simulink model "case8"  (R2024b)
settings: Solver=FixedStepAuto  StartTime=0  StopTime=1  FixedStep=1e-7  RelTol=1e-3
values from neighbouring files (symbols this model uses):
  SG_D_1_D = 0.01056    [IEEE9_case_parameters.m]    (also in case1_parameters.m; case2_parameters.m; case3_parameters.m; case4_parameters.m)
  SG_D_1_EnableSaturation = 0    [IEEE9_case_parameters.m]    (also in case1_parameters.m; case2_parameters.m; case3_parameters.m; case4_parameters.m)
  SG_D_1_f0 = 60    [IEEE9_case_parameters.m]    (also in case1_parameters.m; case2_parameters.m; case3_parameters.m; case4_parameters.m)
  SG_D_1_H = 7.5    [IEEE9_case_parameters.m]    (also in case1_parameters.m; case2_parameters.m; case3_parameters.m; case4_parameters.m)
  SG_D_1_K_A = 20    [IEEE9_case_parameters.m]    (also in case1_parameters.m; case2_parameters.m; case3_parameters.m; case4_parameters.m)
  SG_D_1_K_E = 1.000000e+1    (= 10)    [IEEE9_case_parameters.m]    (also in case1_parameters.m; case2_parameters.m; case3_parameters.m; case4_parameters.m)
  SG_D_1_K_F = 2.363    [IEEE9_case_parameters.m]    (also in case1_parameters.m; case2_parameters.m; case3_parameters.m; case4_parameters.m)
  SG_D_1_K_s = 0.5    [IEEE9_case_parameters.m]    (also in case1_parameters.m = 5; case2_parameters.m = 5; case3_parameters.m = 5; case4_parameters.m = 5)
  SG_D_1_R_a = 0.001088    [IEEE9_case_parameters.m]    (also in case1_parameters.m; case2_parameters.m; case3_parameters.m; case4_parameters.m)
  SG_D_1_S_A = 1    [IEEE9_case_parameters.m]    (also in case1_parameters.m; case2_parameters.m; case3_parameters.m; case4_parameters.m)
  SG_D_1_S_B = 0.103    [IEEE9_case_parameters.m]    (also in case1_parameters.m; case2_parameters.m; case3_parameters.m; case4_parameters.m)
  SG_D_1_S_N = 10.659857    [IEEE9_case_parameters.m]    (also in case1_parameters.m; case2_parameters.m; case3_parameters.m; case4_parameters.m)
  SG_D_1_SpeedPara = 200    [IEEE9_case_parameters.m]    (also in case1_parameters.m; case2_parameters.m; case3_parameters.m; case4_parameters.m)
  SG_D_1_T_0 = 0.720173    [IEEE9_case_parameters.m]    (also in case1_parameters.m = 0.755522; case2_parameters.m = 0.808931; case3_parameters.m = 0.869402; case4_parameters.m = 0.729316)
  SG_D_1_T_1 = 0.3    [IEEE9_case_parameters.m]    (also in case1_parameters.m; case2_parameters.m; case3_parameters.m; case4_parameters.m)
  SG_D_1_T_2 = 0.05    [IEEE9_case_parameters.m]    (also in case1_parameters.m; case2_parameters.m; case3_parameters.m; case4_parameters.m)
  SG_D_1_T_3 = 0.02    [IEEE9_case_parameters.m]    (also in case1_parameters.m; case2_parameters.m; case3_parameters.m; case4_parameters.m)
  SG_D_1_T_4 = 0.005    [IEEE9_case_parameters.m]    (also in case1_parameters.m; case2_parameters.m; case3_parameters.m; case4_parameters.m)
  SG_D_1_T_A = 0.02    [IEEE9_case_parameters.m]    (also in case1_parameters.m; case2_parameters.m; case3_parameters.m; case4_parameters.m)
  SG_D_1_T_dd = 8.000000e+0    (= 8)    [IEEE9_case_parameters.m]    (also in case1_parameters.m; case2_parameters.m; case3_parameters.m; case4_parameters.m)
  SG_D_1_T_ddd = 0.04    [IEEE9_case_parameters.m]    (also in case1_parameters.m; case2_parameters.m; case3_parameters.m; case4_parameters.m)
  SG_D_1_T_E = 0.314    [IEEE9_case_parameters.m]    (also in case1_parameters.m; case2_parameters.m; case3_parameters.m; case4_parameters.m)
  SG_D_1_T_F = 0.35    [IEEE9_case_parameters.m]    (also in case1_parameters.m; case2_parameters.m; case3_parameters.m; case4_parameters.m)
  SG_D_1_T_qd = 0.8    [IEEE9_case_parameters.m]    (also in case1_parameters.m; case2_parameters.m; case3_parameters.m; case4_parameters.m)
  SG_D_1_T_qdd = 0.02    [IEEE9_case_parameters.m]    (also in case1_parameters.m; case2_parameters.m; case3_parameters.m; case4_parameters.m)
  SG_D_1_T_speed = 0.1    [IEEE9_case_parameters.m]    (also in case1_parameters.m = 200; case2_parameters.m = 200; case3_parameters.m = 200; case4_parameters.m = 200)
  SG_D_1_T_w = 0.5    [IEEE9_case_parameters.m]    (also in case1_parameters.m; case2_parameters.m; case3_parameters.m; case4_parameters.m)
  SG_D_1_V_ref = 1.990276    [IEEE9_case_parameters.m]    (also in case1_parameters.m = 2.042296; case2_parameters.m = 2.051388; case3_parameters.m = 2.089584; case4_parameters.m = 2.01845)
  SG_D_1_w_ref = 376.991118    [IEEE9_case_parameters.m]    (also in case1_parameters.m; case2_parameters.m; case3_parameters.m; case4_parameters.m)
  SG_D_1_wb = 6.000000e+1    (= 60)    [IEEE9_case_parameters.m]    (also in case1_parameters.m; case2_parameters.m; case3_parameters.m; case4_parameters.m)
  SG_D_1_x_d = 1.9    [IEEE9_case_parameters.m]    (also in case1_parameters.m; case2_parameters.m; case3_parameters.m; case4_parameters.m)
  SG_D_1_x_dd = 0.302    [IEEE9_case_parameters.m]    (also in case1_parameters.m; case2_parameters.m; case3_parameters.m; case4_parameters.m)
  SG_D_1_x_ddd = 0.204    [IEEE9_case_parameters.m]    (also in case1_parameters.m; case2_parameters.m; case3_parameters.m; case4_parameters.m)
  SG_D_1_x_l = 0.05    [IEEE9_case_parameters.m]    (also in case1_parameters.m; case2_parameters.m; case3_parameters.m; case4_parameters.m)
  SG_D_1_x_q = 1.3    [IEEE9_case_parameters.m]    (also in case1_parameters.m; case2_parameters.m; case3_parameters.m; case4_parameters.m)
  SG_D_1_x_qd = 0.5    [IEEE9_case_parameters.m]    (also in case1_parameters.m; case2_parameters.m; case3_parameters.m; case4_parameters.m)
  SG_D_1_x_qdd = 0.3    [IEEE9_case_parameters.m]    (also in case1_parameters.m; case2_parameters.m; case3_parameters.m; case4_parameters.m)
  SG_D_2_D = 0.02    [IEEE9_case_parameters.m]    (also in case1_parameters.m; case2_parameters.m; case3_parameters.m; case4_parameters.m)
  SG_D_2_EnableSaturation = 0    [IEEE9_case_parameters.m]    (also in case1_parameters.m; case2_parameters.m; case3_parameters.m; case4_parameters.m)
  SG_D_2_f0 = 60    [IEEE9_case_parameters.m]    (also in case1_parameters.m; case2_parameters.m; case3_parameters.m; case4_parameters.m)
  SG_D_2_H = 8.000000e+0    (= 8)    [IEEE9_case_parameters.m]    (also in case1_parameters.m; case2_parameters.m; case3_parameters.m; case4_parameters.m)
  SG_D_2_K_A = 20    [IEEE9_case_parameters.m]    (also in case1_parameters.m; case2_parameters.m; case3_parameters.m; case4_parameters.m)
  SG_D_2_K_E = 1.000000e+1    (= 10)    [IEEE9_case_parameters.m]    (also in case1_parameters.m; case2_parameters.m; case3_parameters.m; case4_parameters.m)
  SG_D_2_K_F = 2.363    [IEEE9_case_parameters.m]    (also in case1_parameters.m; case2_parameters.m; case3_parameters.m; case4_parameters.m)
  SG_D_2_K_s = 0.5    [IEEE9_case_parameters.m]    (also in case1_parameters.m = 4; case2_parameters.m = 4; case3_parameters.m = 4; case4_parameters.m = 4)
  SG_D_2_R_a = 0.001088    [IEEE9_case_parameters.m]    (also in case1_parameters.m; case2_parameters.m; case3_parameters.m; case4_parameters.m)
  SG_D_2_S_A = 1    [IEEE9_case_parameters.m]    (also in case1_parameters.m; case2_parameters.m; case3_parameters.m; case4_parameters.m)
  SG_D_2_S_B = 0.103    [IEEE9_case_parameters.m]    (also in case1_parameters.m; case2_parameters.m; case3_parameters.m; case4_parameters.m)
  SG_D_2_S_N = 10.659857    [IEEE9_case_parameters.m]    (also in case1_parameters.m; case2_parameters.m; case3_parameters.m; case4_parameters.m)
  SG_D_2_SpeedPara = 200    [IEEE9_case_parameters.m]    (also in case1_parameters.m; case2_parameters.m; case3_parameters.m; case4_parameters.m)
  SG_D_2_T_0 = 1.632913    [IEEE9_case_parameters.m]    (also in case1_parameters.m = 1.632925; case2_parameters.m = 1.632915; case3_parameters.m = 1.632914; case4_parameters.m = 1.632927)
  SG_D_2_T_1 = 0.2    [IEEE9_case_parameters.m]    (also in case1_parameters.m; case2_parameters.m; case3_parameters.m; case4_parameters.m)
  SG_D_2_T_2 = 0.05    [IEEE9_case_parameters.m]    (also in case1_parameters.m; case2_parameters.m; case3_parameters.m; case4_parameters.m)
  SG_D_2_T_3 = 0.02    [IEEE9_case_parameters.m]    (also in case1_parameters.m; case2_parameters.m; case3_parameters.m; case4_parameters.m)
  SG_D_2_T_4 = 0.005    [IEEE9_case_parameters.m]    (also in case1_parameters.m; case2_parameters.m; case3_parameters.m; case4_parameters.m)
  SG_D_2_T_A = 0.02    [IEEE9_case_parameters.m]    (also in case1_parameters.m; case2_parameters.m; case3_parameters.m; case4_parameters.m)
  SG_D_2_T_dd = 7.9    [IEEE9_case_parameters.m]    (also in case1_parameters.m; case2_parameters.m; case3_parameters.m; case4_parameters.m)
  SG_D_2_T_ddd = 0.04    [IEEE9_case_parameters.m]    (also in case1_parameters.m; case2_parameters.m; case3_parameters.m; case4_parameters.m)
  SG_D_2_T_E = 0.314    [IEEE9_case_parameters.m]    (also in case1_parameters.m; case2_parameters.m; case3_parameters.m; case4_parameters.m)
  SG_D_2_T_F = 0.35    [IEEE9_case_parameters.m]    (also in case1_parameters.m; case2_parameters.m; case3_parameters.m; case4_parameters.m)
  SG_D_2_T_qd = 0.8    [IEEE9_case_parameters.m]    (also in case1_parameters.m; case2_parameters.m; case3_parameters.m; case4_parameters.m)
  SG_D_2_T_qdd = 0.015    [IEEE9_case_parameters.m]    (also in case1_parameters.m; case2_parameters.m; case3_parameters.m; case4_parameters.m)
  SG_D_2_T_speed = 0.1    [IEEE9_case_parameters.m]    (also in case1_parameters.m = 150; case2_parameters.m = 150; case3_parameters.m = 150; case4_parameters.m = 150)
  SG_D_2_T_w = 0.35    [IEEE9_case_parameters.m]    (also in case1_parameters.m; case2_parameters.m; case3_parameters.m; case4_parameters.m)
  SG_D_2_V_ref = 2.58547    [IEEE9_case_parameters.m]    (also in case1_parameters.m = 2.597896; case2_parameters.m = 2.587136; case3_parameters.m = 2.586042; case4_parameters.m = 2.599679)
  SG_D_2_w_ref = 376.991118    [IEEE9_case_parameters.m]    (also in case1_parameters.m; case2_parameters.m; case3_parameters.m; case4_parameters.m)
  SG_D_2_wb = 6.000000e+1    (= 60)    [IEEE9_case_parameters.m]    (also in case1_parameters.m; case2_parameters.m; case3_parameters.m; case4_parameters.m)
  SG_D_2_x_d = 1.8    [IEEE9_case_parameters.m]    (also in case1_parameters.m; case2_parameters.m; case3_parameters.m; case4_parameters.m)
  SG_D_2_x_dd = 0.302    [IEEE9_case_parameters.m]    (also in case1_parameters.m; case2_parameters.m; case3_parameters.m; case4_parameters.m)
  SG_D_2_x_ddd = 0.204    [IEEE9_case_parameters.m]    (also in case1_parameters.m; case2_parameters.m; case3_parameters.m; case4_parameters.m)
  SG_D_2_x_l = 0.05    [IEEE9_case_parameters.m]    (also in case1_parameters.m; case2_parameters.m; case3_parameters.m; case4_parameters.m)
  SG_D_2_x_q = 1.25    [IEEE9_case_parameters.m]    (also in case1_parameters.m; case2_parameters.m; case3_parameters.m; case4_parameters.m)
  SG_D_2_x_qd = 0.5    [IEEE9_case_parameters.m]    (also in case1_parameters.m; case2_parameters.m; case3_parameters.m; case4_parameters.m)
  SG_D_2_x_qdd = 0.3    [IEEE9_case_parameters.m]    (also in case1_parameters.m; case2_parameters.m; case3_parameters.m; case4_parameters.m)
  SG_D_3_D = 0.02    [IEEE9_case_parameters.m]    (also in case1_parameters.m; case2_parameters.m; case3_parameters.m; case4_parameters.m)
  SG_D_3_EnableSaturation = 0    [IEEE9_case_parameters.m]    (also in case1_parameters.m; case2_parameters.m; case3_parameters.m; case4_parameters.m)
  SG_D_3_f0 = 60    [IEEE9_case_parameters.m]    (also in case1_parameters.m; case2_parameters.m; case3_parameters.m; case4_parameters.m)
  SG_D_3_H = 7.7    [IEEE9_case_parameters.m]    (also in case1_parameters.m; case2_parameters.m; case3_parameters.m; case4_parameters.m)
  SG_D_3_K_A = 20    [IEEE9_case_parameters.m]    (also in case1_parameters.m; case2_parameters.m; case3_parameters.m; case4_parameters.m)
  SG_D_3_K_E = 1.000000e+1    (= 10)    [IEEE9_case_parameters.m]    (also in case1_parameters.m; case2_parameters.m; case3_parameters.m; case4_parameters.m)
  SG_D_3_K_F = 2.363    [IEEE9_case_parameters.m]    (also in case1_parameters.m; case2_parameters.m; case3_parameters.m; case4_parameters.m)
  SG_D_3_K_s = 0.2    [IEEE9_case_parameters.m]    (also in case1_parameters.m = 2; case2_parameters.m = 2; case3_parameters.m = 2; case4_parameters.m = 2)
  SG_D_3_R_a = 0.001088    [IEEE9_case_parameters.m]    (also in case1_parameters.m; case2_parameters.m; case3_parameters.m; case4_parameters.m)
  SG_D_3_S_A = 1    [IEEE9_case_parameters.m]    (also in case1_parameters.m; case2_parameters.m; case3_parameters.m; case4_parameters.m)
  SG_D_3_S_B = 0.103    [IEEE9_case_parameters.m]    (also in case1_parameters.m; case2_parameters.m; case3_parameters.m; case4_parameters.m)
  SG_D_3_S_N = 10.659857    [IEEE9_case_parameters.m]    (also in case1_parameters.m; case2_parameters.m; case3_parameters.m; case4_parameters.m)
  SG_D_3_SpeedPara = 200    [IEEE9_case_parameters.m]    (also in case1_parameters.m; case2_parameters.m; case3_parameters.m; case4_parameters.m)
  SG_D_3_T_0 = 0.850788    [IEEE9_case_parameters.m]    (also in case1_parameters.m = 0.850786; case2_parameters.m = 0.850787; case3_parameters.m; case4_parameters.m = 0.850786)
  SG_D_3_T_1 = 0.2    [IEEE9_case_parameters.m]    (also in case1_parameters.m; case2_parameters.m; case3_parameters.m; case4_parameters.m)
  SG_D_3_T_2 = 0.05    [IEEE9_case_parameters.m]    (also in case1_parameters.m; case2_parameters.m; case3_parameters.m; case4_parameters.m)
  SG_D_3_T_3 = 0.02    [IEEE9_case_parameters.m]    (also in case1_parameters.m; case2_parameters.m; case3_parameters.m; case4_parameters.m)
  SG_D_3_T_4 = 0.005    [IEEE9_case_parameters.m]    (also in case1_parameters.m; case2_parameters.m; case3_parameters.m; case4_parameters.m)
  SG_D_3_T_A = 0.02    [IEEE9_case_parameters.m]    (also in case1_parameters.m; case2_parameters.m; case3_parameters.m; case4_parameters.m)
  SG_D_3_T_dd = 8.1    [IEEE9_case_parameters.m]    (also in case1_parameters.m; case2_parameters.m; case3_parameters.m; case4_parameters.m)
  SG_D_3_T_ddd = 0.04    [IEEE9_case_parameters.m]    (also in case1_parameters.m; case2_parameters.m; case3_parameters.m; case4_parameters.m)
  SG_D_3_T_E = 0.314    [IEEE9_case_parameters.m]    (also in case1_parameters.m; case2_parameters.m; case3_parameters.m; case4_parameters.m)
  SG_D_3_T_F = 0.35    [IEEE9_case_parameters.m]    (also in case1_parameters.m; case2_parameters.m; case3_parameters.m; case4_parameters.m)
  SG_D_3_T_qd = 0.8    [IEEE9_case_parameters.m]    (also in case1_parameters.m; case2_parameters.m; case3_parameters.m; case4_parameters.m)
  SG_D_3_T_qdd = 0.015    [IEEE9_case_parameters.m]    (also in case1_parameters.m; case2_parameters.m; case3_parameters.m; case4_parameters.m)
  SG_D_3_T_speed = 0.1    [IEEE9_case_parameters.m]    (also in case1_parameters.m = 180; case2_parameters.m = 180; case3_parameters.m = 180; case4_parameters.m = 180)
  SG_D_3_T_w = 0.4    [IEEE9_case_parameters.m]    (also in case1_parameters.m; case2_parameters.m; case3_parameters.m; case4_parameters.m)
  SG_D_3_V_ref = 1.892727    [IEEE9_case_parameters.m]    (also in case1_parameters.m = 1.906439; case2_parameters.m = 1.895535; case3_parameters.m = 1.892105; case4_parameters.m = 1.906598)
  SG_D_3_w_ref = 376.991118    [IEEE9_case_parameters.m]    (also in case1_parameters.m; case2_parameters.m; case3_parameters.m; case4_parameters.m)
  SG_D_3_wb = 6.000000e+1    (= 60)    [IEEE9_case_parameters.m]    (also in case1_parameters.m; case2_parameters.m; case3_parameters.m; case4_parameters.m)
  SG_D_3_x_d = 1.85    [IEEE9_case_parameters.m]    (also in case1_parameters.m; case2_parameters.m; case3_parameters.m; case4_parameters.m)
  SG_D_3_x_dd = 0.302    [IEEE9_case_parameters.m]    (also in case1_parameters.m; case2_parameters.m; case3_parameters.m; case4_parameters.m)
  SG_D_3_x_ddd = 0.204    [IEEE9_case_parameters.m]    (also in case1_parameters.m; case2_parameters.m; case3_parameters.m; case4_parameters.m)
  SG_D_3_x_l = 0.05    [IEEE9_case_parameters.m]    (also in case1_parameters.m; case2_parameters.m; case3_parameters.m; case4_parameters.m)
  SG_D_3_x_q = 1.2    [IEEE9_case_parameters.m]    (also in case1_parameters.m; case2_parameters.m; case3_parameters.m; case4_parameters.m)
  SG_D_3_x_qd = 0.5    [IEEE9_case_parameters.m]    (also in case1_parameters.m; case2_parameters.m; case3_parameters.m; case4_parameters.m)
  SG_D_3_x_qdd = 0.3    [IEEE9_case_parameters.m]    (also in case1_parameters.m; case2_parameters.m; case3_parameters.m; case4_parameters.m)
(part 10 of 12)

== system case8/SG_D_3/d_R_f_SG_D_3_block ==
  note: d_R_f_SG_D_3 in case8
      | $-\frac{R_{f,\mathrm{SG},D,3}-\frac{E_{\mathrm{fd},\mathrm{SG},D,3}\,K_{F}}{T_{F}}}{T_{F}}$
      | Automatically generated on 2025-10-31 19:30:15 .
  State_E_fd_SG_D_3_84f8d : Inport
  State_R_f_SG_D_3_58aed : Inport  Port=2
  Constant_K_F_20094 : Constant  Value=K_F
  Constant_T_F_9f9dd : Constant  Value=T_F
  Constant_T_F_ee7b0 : Constant  Value=T_F
  Divide_112f1 : Product  Inputs=*/
  Divide_9077d : Product  Inputs=*/
  Product_25227 : Product
  Subtract_40c17 : Sum  Inputs=+-
  Blockout_d_R_f_SG_D_3_82a7f : Outport
  wires:
  State_E_fd_SG_D_3_84f8d/1 -> Product_25227/1
  Constant_T_F_ee7b0/1 -> Divide_112f1/2
  Constant_K_F_20094/1 -> Product_25227/2
  Product_25227/1 -> Divide_112f1/1
  Divide_112f1/1 -> Subtract_40c17/1
  State_R_f_SG_D_3_58aed/1 -> Subtract_40c17/2
  Subtract_40c17/1 -> Divide_9077d/1
  Constant_T_F_9f9dd/1 -> Divide_9077d/2
  Divide_9077d/1 -> Blockout_d_R_f_SG_D_3_82a7f/1

== system case8/SG_D_3/d_T_m_SG_D_3_block ==
  note: d_T_m_SG_D_3 in case8
      | $-\frac{T_{m,\mathrm{SG},D,3}-T_{0}+\frac{\mathrm{SpeedPara}\,\left(w_{\mathrm{SG},D,3}-w_{\mathrm{ref}}\right)}{2\,f_{0}\,\pi }}{T_{\mathrm{speed}}}$
      | Automatically generated on 2025-10-31 19:30:13 .
  State_w_SG_D_3_a06af : Inport
  State_T_m_SG_D_3_22a90 : Inport  Port=2
  Add_c0c64 : Sum
  Add_d464c : Sum
  Constant_-1_5bfeb : Constant  Value=-1
  Constant_2.0_e0f47 : Constant  Value=2.0
  Constant_SpeedPara_10a21 : Constant  Value=SpeedPara
  Constant_T_0_56f13 : Constant  Value=T_0
  Constant_T_speed_ee43e : Constant  Value=T_speed
  Constant_f0_46ba4 : Constant  Value=f0
  Constant_pi_74b3a : Constant  Value=pi
  Constant_w_ref_43c65 : Constant  Value=w_ref
  Divide_22875 : Product  Inputs=*/
  Divide_477d5 : Product  Inputs=*/
  Product_4319f : Product
  Product_c0b05 : Product
  Product_c9b07 : Product
  Product_f2fe5 : Product
  Subtract_bdcef : Sum  Inputs=+-
  Blockout_d_T_m_SG_D_3_869a6 : Outport
  wires:
  Constant_SpeedPara_10a21/1 -> Product_c0b05/1
  Constant_-1_5bfeb/1 -> Product_f2fe5/1
  Constant_w_ref_43c65/1 -> Add_d464c/2
  State_w_SG_D_3_a06af/1 -> Product_f2fe5/2
  Constant_2.0_e0f47/1 -> Product_c9b07/1
  Product_f2fe5/1 -> Add_d464c/1
  Constant_pi_74b3a/1 -> Product_c9b07/2
  Add_d464c/1 -> Product_c0b05/2
  Product_c9b07/1 -> Product_4319f/1
  Constant_f0_46ba4/1 -> Product_4319f/2
  Product_c0b05/1 -> Divide_477d5/1
  Product_4319f/1 -> Divide_477d5/2
  Divide_477d5/1 -> Add_c0c64/1
  Constant_T_0_56f13/1 -> Add_c0c64/2
  Add_c0c64/1 -> Subtract_bdcef/1
  State_T_m_SG_D_3_22a90/1 -> Subtract_bdcef/2
  Subtract_bdcef/1 -> Divide_22875/1
  Constant_T_speed_ee43e/1 -> Divide_22875/2
  Divide_22875/1 -> Blockout_d_T_m_SG_D_3_869a6/1

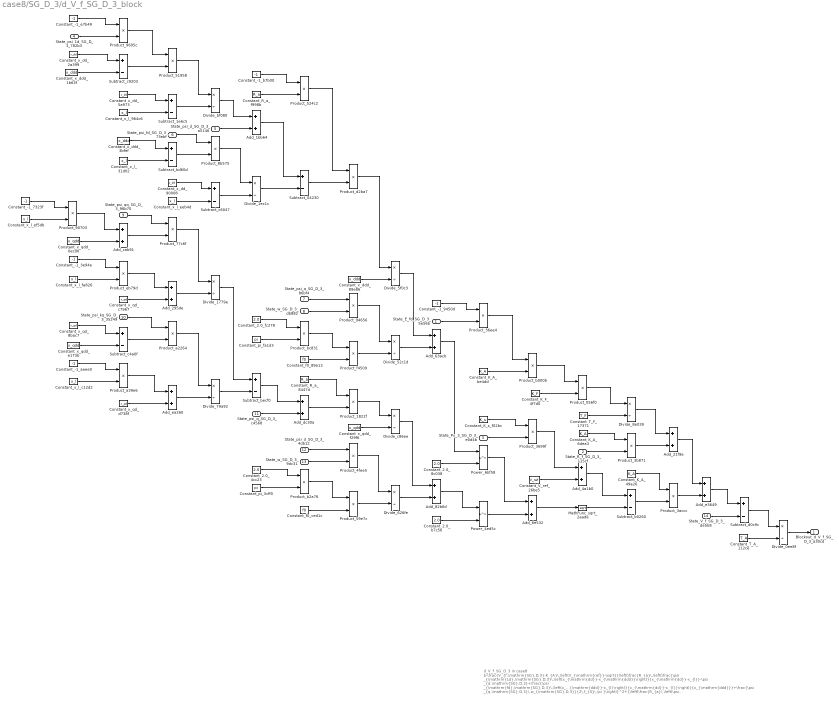
== system case8/SG_D_3/d_V_f_SG_D_3_block ==
  note: d_V_f_SG_D_3 in case8
      | $-\frac{V_{f,\mathrm{SG},D,3}-K_{A}\,\left(V_{\mathrm{ref}}-\sqrt{{\left(\frac{R_{a}\,\left(\frac{\psi _{\mathrm{1d},\mathrm{SG},D,3}\,\left(x_{\mathrm{dd}}-x_{\mathrm{ddd}}\right)}{x_{\mathrm{dd}}-x_{l}}-\psi _{d,\mathrm{SG},D,3}+\frac{\psi _{\mathrm{fd},\mathrm{SG},D,3}\,\left(x_{\mathrm{ddd}}-x_{l}\right)}{x_{\mathrm{dd}}-x_{l}}\right)}{x_{\mathrm{ddd}}}+\frac{\psi _{q,\mathrm{SG},D,3}\,w_{\mathrm{SG},D,3}}{2\,f_{0}\,\pi }\right)}^2+{\left(\frac{R_{a}\,\left(\psi _{q,\mathrm{SG},D,3}+\frac{\psi _{\mathrm{gq},\mathrm{SG},D,3}\,\left(x_{l}-x_{\mathrm{qdd}}\right)}{x_{l}-x_{\mathrm{qd}}}+\frac{\psi _{\mathrm{kq},\mathrm{SG},D,3}\,\left(x_{\mathrm{qd}}-x_{\mathrm{qdd}}\right)}{x_{l}-x_{\mathrm{qd}}}\right)}{x_{\mathrm{qdd}}}+\frac{\psi _{d,\mathrm{SG},D,3}\,w_{\mathrm{SG},D,3}}{2\,f_{0}\,\pi }\right)}^2}+K_{s}\,\mathrm{Px}_{3,\mathrm{SG},D,3}\right)-K_{A}\,R_{f,\mathrm{SG},D,3}+\frac{E_{\mathrm{fd},\mathrm{SG},D,3}\,K_{A}\,K_{F}}{T_{F}}}{T_{A}}$
      | Automatically generated on 2025-10-31 19:30:15 .
  State_E_fd_SG_D_3_5e56b : Inport
  State_R_f_SG_D_3_115cf : Inport  Port=2
  State_Px_3_SG_D_3_e0d4b : Inport  Port=3
  State_psi_1d_SG_D_3_782b3 : Inport  Port=4
  State_psi_d_SG_D_3_a5146 : Inport  Port=5
  State_psi_fd_SG_D_3_73ebf : Inport  Port=6
  State_psi_q_SG_D_3_86bf4 : Inport  Port=7
  State_w_SG_D_3_db882 : Inport  Port=8
  State_psi_gq_SG_D_3_96b70 : Inport  Port=9
  State_psi_kq_SG_D_3_35249 : Inport  Port=10
  State_psi_q_SG_D_3_c4568 : Inport  Port=11
  State_psi_d_SG_D_3_4db12 : Inport  Port=12
  State_w_SG_D_3_9dc31 : Inport  Port=13
  State_V_f_SG_D_3_de5b8 : Inport  Port=14
  Add_1bb64 : Sum
  Add_21f9e : Sum
  Add_295de : Sum
  Add_4a1b0 : Sum
  Add_63acb : Sum
  Add_6e532 : Sum
  Add_82b6d : Sum
  Add_cab91 : Sum
  Add_dc30a : Sum
  Add_e3649 : Sum
  Add_ea260 : Sum
  Constant_-1_3e94e : Constant  Value=-1
  Constant_-1_7323f : Constant  Value=-1
  Constant_-1_9450d : Constant  Value=-1
  Constant_-1_aeee0 : Constant  Value=-1
  Constant_-1_b7b00 : Constant  Value=-1
  Constant_-1_e7b49 : Constant  Value=-1
  Constant_2.0_4cc23 : Constant  Value=2.0
  Constant_2.0_8c038 : Constant  Value=2.0
  Constant_2.0_b7c56 : Constant  Value=2.0
  Constant_2.0_fc278 : Constant  Value=2.0
  Constant_K_A_49a26 : Constant  Value=K_A
  Constant_K_A_6dea3 : Constant  Value=K_A
  Constant_K_A_be4dd : Constant  Value=K_A
  Constant_K_F_4f7d0 : Constant  Value=K_F
  Constant_K_s_f02bc : Constant  Value=K_s
  Constant_R_a_8447d : Constant  Value=R_a
  Constant_R_a_f998b : Constant  Value=R_a
  Constant_T_A_112ce : Constant  Value=T_A
  Constant_T_F_17371 : Constant  Value=T_F
  Constant_V_ref_26be5 : Constant  Value=V_ref
  Constant_f0_89e13 : Constant  Value=f0
  Constant_f0_ced1c : Constant  Value=f0
  Constant_pi_3cff0 : Constant  Value=pi
  Constant_pi_fa1d3 : Constant  Value=pi
  Constant_x_dd_2a399 : Constant  Value=x_dd
  Constant_x_dd_5a973 : Constant  Value=x_dd
  Constant_x_dd_90008 : Constant  Value=x_dd
  Constant_x_ddd_1b63f : Constant  Value=x_ddd
  Constant_x_ddd_3bfef : Constant  Value=x_ddd
  Constant_x_ddd_89e86 : Constant  Value=x_ddd
  Constant_x_l_31d02 : Constant  Value=x_l
  Constant_x_l_964c6 : Constant  Value=x_l
  Constant_x_l_c12d2 : Constant  Value=x_l
  Constant_x_l_eeb4d : Constant  Value=x_l
  Constant_x_l_ef5db : Constant  Value=x_l
  Constant_x_l_fa826 : Constant  Value=x_l
  Constant_x_qd_8bac7 : Constant  Value=x_qd
  Constant_x_qd_c7967 : Constant  Value=x_qd
  Constant_x_qd_d738f : Constant  Value=x_qd
  Constant_x_qdd_0ecd0 : Constant  Value=x_qdd
  Constant_x_qdd_e173b : Constant  Value=x_qdd
  Constant_x_qdd_f29f6 : Constant  Value=x_qdd
  Divide_0ee8f : Product  Inputs=*/
  Divide_1779e : Product  Inputs=*/
  Divide_1ec1c : Product  Inputs=*/
  Divide_52c1d : Product  Inputs=*/
  Divide_5f0c3 : Product  Inputs=*/
  Divide_626fe : Product  Inputs=*/
  Divide_79a92 : Product  Inputs=*/
  Divide_8e039 : Product  Inputs=*/
  Divide_bf080 : Product  Inputs=*/
  Divide_c86ee : Product  Inputs=*/
  MathFunc_sqrt_2aade : Sqrt
  Power_4ed5c : Math  Operator=pow
  Power_6bf58 : Math  Operator=pow
  Product_056f0 : Product
  Product_1822f : Product
  Product_3699f : Product
  Product_36ee4 : Product
  Product_3accc : Product
  Product_3b871 : Product
  Product_4fee5 : Product
  Product_51958 : Product
  Product_524c2 : Product
  Product_59e7c : Product
  Product_77c6f : Product
  Product_8b575 : Product
  Product_90703 : Product
  Product_94656 : Product
  Product_9695c : Product
  Product_a2264 : Product
  Product_a39e6 : Product
  Product_b000b : Product
  Product_b2a76 : Product
  Product_bc831 : Product
  Product_d2ba7 : Product
  Product_eb79d : Product
  Product_f4509 : Product
  Subtract_04230 : Sum  Inputs=+-
  Subtract_1e6c5 : Sum  Inputs=+-
  Subtract_b0260 : Sum  Inputs=+-
  Subtract_bd60d : Sum  Inputs=+-
  Subtract_becf0 : Sum  Inputs=+-
  Subtract_c4a0f : Sum  Inputs=+-
  Subtract_c6047 : Sum  Inputs=+-
  Subtract_c9203 : Sum  Inputs=+-
  Subtract_d0c9c : Sum  Inputs=+-
  Blockout_d_V_f_SG_D_3_a30cd : Outport
  wires:
  Constant_K_A_6dea3/1 -> Product_3b871/1
  Constant_-1_7323f/1 -> Product_90703/1
  Subtract_bd60d/1 -> Product_8b575/2
  Constant_x_l_ef5db/1 -> Product_90703/2
  Divide_626fe/1 -> Add_82b6d/2
  Constant_-1_e7b49/1 -> Product_9695c/1
  State_psi_1d_SG_D_3_782b3/1 -> Product_9695c/2
  Constant_x_dd_2a399/1 -> Subtract_c9203/1
  Divide_1ec1c/1 -> Subtract_04230/2
  Product_90703/1 -> Add_cab91/1
  Constant_x_qdd_0ecd0/1 -> Add_cab91/2
  Constant_x_ddd_1b63f/1 -> Subtract_c9203/2
  Constant_2.0_b7c56/1 -> Power_4ed5c/2
  Constant_-1_3e94e/1 -> Product_eb79d/1
  Divide_1779e/1 -> Subtract_becf0/1
  Subtract_1e6c5/1 -> Divide_bf080/2
  Constant_x_l_fa826/1 -> Product_eb79d/2
  Constant_x_qd_8bac7/1 -> Subtract_c4a0f/1
  State_w_SG_D_3_db882/1 -> Product_94656/2
  Constant_x_qdd_e173b/1 -> Subtract_c4a0f/2
  Constant_2.0_fc278/1 -> Product_bc831/1
  Constant_-1_aeee0/1 -> Product_a39e6/1
  Constant_pi_fa1d3/1 -> Product_bc831/2
  Add_1bb64/1 -> Subtract_04230/1
  Constant_x_l_c12d2/1 -> Product_a39e6/2
  Product_9695c/1 -> Product_51958/1
  Subtract_c9203/1 -> Product_51958/2
  Constant_2.0_4cc23/1 -> Product_b2a76/1
  Constant_x_dd_5a973/1 -> Subtract_1e6c5/1
  Constant_pi_3cff0/1 -> Product_b2a76/2
  Constant_x_l_964c6/1 -> Subtract_1e6c5/2
  Constant_x_ddd_3bfef/1 -> Subtract_bd60d/1
  Constant_x_l_31d02/1 -> Subtract_bd60d/2
  State_psi_gq_SG_D_3_96b70/1 -> Product_77c6f/1
  Constant_x_l_eeb4d/1 -> Subtract_c6047/2
  Add_cab91/1 -> Product_77c6f/2
  Product_eb79d/1 -> Add_295de/1
  Product_77c6f/1 -> Divide_1779e/1
  Constant_x_qd_c7967/1 -> Add_295de/2
  State_psi_kq_SG_D_3_35249/1 -> Product_a2264/1
  State_psi_q_SG_D_3_86bf4/1 -> Product_94656/1
  Add_63acb/1 -> Power_6bf58/1
  Subtract_c4a0f/1 -> Product_a2264/2
  Constant_f0_89e13/1 -> Product_f4509/2
  Product_bc831/1 -> Product_f4509/1
  Constant_x_qd_d738f/1 -> Add_ea260/2
  Product_a39e6/1 -> Add_ea260/1
  Product_51958/1 -> Divide_bf080/1
  State_psi_fd_SG_D_3_73ebf/1 -> Product_8b575/1
  Constant_x_dd_90008/1 -> Subtract_c6047/1
  Add_295de/1 -> Divide_1779e/2
  Add_6e532/1 -> MathFunc_sqrt_2aade/1
  Product_a2264/1 -> Divide_79a92/1
  Add_ea260/1 -> Divide_79a92/2
  Product_524c2/1 -> Product_d2ba7/1
  Divide_bf080/1 -> Add_1bb64/1
  Add_4a1b0/1 -> Subtract_b0260/1
  State_psi_d_SG_D_3_a5146/1 -> Add_1bb64/2
  Product_8b575/1 -> Divide_1ec1c/1
  Subtract_c6047/1 -> Divide_1ec1c/2
  MathFunc_sqrt_2aade/1 -> Subtract_b0260/2
  Divide_79a92/1 -> Subtract_becf0/2
  Constant_-1_b7b00/1 -> Product_524c2/1
  Constant_R_a_f998b/1 -> Product_524c2/2
  Subtract_becf0/1 -> Add_dc30a/1
  State_psi_q_SG_D_3_c4568/1 -> Add_dc30a/2
  Subtract_04230/1 -> Product_d2ba7/2
  Constant_R_a_8447d/1 -> Product_1822f/1
  Add_dc30a/1 -> Product_1822f/2
  State_psi_d_SG_D_3_4db12/1 -> Product_4fee5/1
  State_w_SG_D_3_9dc31/1 -> Product_4fee5/2
  Product_b2a76/1 -> Product_59e7c/1
  Constant_f0_ced1c/1 -> Product_59e7c/2
  Product_d2ba7/1 -> Divide_5f0c3/1
  Constant_x_ddd_89e86/1 -> Divide_5f0c3/2
  Product_94656/1 -> Divide_52c1d/1
  Product_f4509/1 -> Divide_52c1d/2
  Product_1822f/1 -> Divide_c86ee/1
  Constant_x_qdd_f29f6/1 -> Divide_c86ee/2
  Product_4fee5/1 -> Divide_626fe/1
  Product_59e7c/1 -> Divide_626fe/2
  Divide_5f0c3/1 -> Add_63acb/1
  Divide_52c1d/1 -> Add_63acb/2
  Divide_c86ee/1 -> Add_82b6d/1
  Constant_-1_9450d/1 -> Product_36ee4/1
  State_E_fd_SG_D_3_5e56b/1 -> Product_36ee4/2
  Constant_2.0_8c038/1 -> Power_6bf58/2
  Add_82b6d/1 -> Power_4ed5c/1
  Product_36ee4/1 -> Product_b000b/1
  Constant_K_A_be4dd/1 -> Product_b000b/2
  Constant_K_s_f02bc/1 -> Product_3699f/1
  State_Px_3_SG_D_3_e0d4b/1 -> Product_3699f/2
  Power_6bf58/1 -> Add_6e532/1
  Power_4ed5c/1 -> Add_6e532/2
  Product_b000b/1 -> Product_056f0/1
  Constant_K_F_4f7d0/1 -> Product_056f0/2
  Product_3699f/1 -> Add_4a1b0/1
  Constant_V_ref_26be5/1 -> Add_4a1b0/2
  Product_056f0/1 -> Divide_8e039/1
  Constant_T_F_17371/1 -> Divide_8e039/2
  Add_e3649/1 -> Subtract_d0c9c/1
  State_R_f_SG_D_3_115cf/1 -> Product_3b871/2
  Divide_8e039/1 -> Add_21f9e/1
  Product_3b871/1 -> Add_21f9e/2
  Constant_K_A_49a26/1 -> Product_3accc/1
  Subtract_b0260/1 -> Product_3accc/2
  Add_21f9e/1 -> Add_e3649/1
  Product_3accc/1 -> Add_e3649/2
  State_V_f_SG_D_3_de5b8/1 -> Subtract_d0c9c/2
  Subtract_d0c9c/1 -> Divide_0ee8f/1
  Constant_T_A_112ce/1 -> Divide_0ee8f/2
  Divide_0ee8f/1 -> Blockout_d_V_f_SG_D_3_a30cd/1

== system case8/SG_D_3/d_psi_1d_SG_D_3_block ==
  note: d_psi_1d_SG_D_3 in case8
      | $-\frac{\psi _{\mathrm{1d},\mathrm{SG},D,3}-\psi _{\mathrm{fd},\mathrm{SG},D,3}+\frac{\left(x_{\mathrm{dd}}-x_{l}\right)\,\left(\frac{\psi _{\mathrm{1d},\mathrm{SG},D,3}\,\left(x_{\mathrm{dd}}-x_{\mathrm{ddd}}\right)}{x_{\mathrm{dd}}-x_{l}}-\psi _{d,\mathrm{SG},D,3}+\frac{\psi _{\mathrm{fd},\mathrm{SG},D,3}\,\left(x_{\mathrm{ddd}}-x_{l}\right)}{x_{\mathrm{dd}}-x_{l}}\right)}{x_{\mathrm{ddd}}}}{T_{\mathrm{ddd}}}$
      | Automatically generated on 2025-10-31 19:30:08 .
  State_psi_1d_SG_D_3_f33a6 : Inport
  State_psi_fd_SG_D_3_35873 : Inport  Port=2
  State_psi_1d_SG_D_3_8c42f : Inport  Port=3
  State_psi_d_SG_D_3_558ca : Inport  Port=4
  State_psi_fd_SG_D_3_d2e28 : Inport  Port=5
  Add_ac568 : Sum
  Add_bc402 : Sum
  Add_e184c : Sum
  Constant_-1_424bd : Constant  Value=-1
  Constant_-1_f7a49 : Constant  Value=-1
  Constant_T_ddd_8ec66 : Constant  Value=T_ddd
  Constant_x_dd_20ca4 : Constant  Value=x_dd
  Constant_x_dd_7f082 : Constant  Value=x_dd
  Constant_x_dd_9ca1c : Constant  Value=x_dd
  Constant_x_dd_b2aff : Constant  Value=x_dd
  Constant_x_ddd_549c7 : Constant  Value=x_ddd
  Constant_x_ddd_581b3 : Constant  Value=x_ddd
  Constant_x_ddd_d37ef : Constant  Value=x_ddd
  Constant_x_l_06483 : Constant  Value=x_l
  Constant_x_l_224e2 : Constant  Value=x_l
  Constant_x_l_b0529 : Constant  Value=x_l
  Constant_x_l_d376d : Constant  Value=x_l
  Divide_0fc3d : Product  Inputs=*/
  Divide_59545 : Product  Inputs=*/
  Divide_7e259 : Product  Inputs=*/
  Divide_b957c : Product  Inputs=*/
  Product_0f4cf : Product
  Product_11e1d : Product
  Product_1d544 : Product
  Product_3c2fb : Product
  Product_6de9c : Product
  Subtract_36910 : Sum  Inputs=+-
  Subtract_563e3 : Sum  Inputs=+-
  Subtract_8d0e8 : Sum  Inputs=+-
  Subtract_aa4bb : Sum  Inputs=+-
  Subtract_c19c3 : Sum  Inputs=+-
  Subtract_d1c76 : Sum  Inputs=+-
  Blockout_d_psi_1d_SG_D_3_b77c8 : Outport
  wires:
  Divide_7e259/1 -> Add_bc402/1
  Subtract_aa4bb/1 -> Product_3c2fb/2
  Constant_-1_f7a49/1 -> Product_0f4cf/1
  Constant_x_dd_7f082/1 -> Subtract_c19c3/1
  State_psi_1d_SG_D_3_8c42f/1 -> Product_0f4cf/2
  Product_0f4cf/1 -> Product_3c2fb/1
  Constant_x_dd_9ca1c/1 -> Subtract_aa4bb/1
  Constant_x_ddd_581b3/1 -> Subtract_aa4bb/2
  Constant_x_l_224e2/1 -> Subtract_c19c3/2
  Constant_x_ddd_d37ef/1 -> Subtract_563e3/1
  Divide_0fc3d/1 -> Blockout_d_psi_1d_SG_D_3_b77c8/1
  Constant_x_l_d376d/1 -> Subtract_563e3/2
  Product_3c2fb/1 -> Divide_7e259/1
  Subtract_c19c3/1 -> Divide_7e259/2
  State_psi_fd_SG_D_3_d2e28/1 -> Product_1d544/1
  Subtract_563e3/1 -> Product_1d544/2
  Constant_x_dd_20ca4/1 -> Subtract_8d0e8/1
  Constant_x_l_06483/1 -> Subtract_8d0e8/2
  State_psi_d_SG_D_3_558ca/1 -> Add_bc402/2
  Product_1d544/1 -> Divide_b957c/1
  Subtract_8d0e8/1 -> Divide_b957c/2
  Constant_x_dd_b2aff/1 -> Subtract_36910/1
  Constant_x_l_b0529/1 -> Subtract_36910/2
  Add_bc402/1 -> Subtract_d1c76/1
  Divide_b957c/1 -> Subtract_d1c76/2
  Constant_-1_424bd/1 -> Product_11e1d/1
  State_psi_1d_SG_D_3_f33a6/1 -> Product_11e1d/2
  State_psi_fd_SG_D_3_35873/1 -> Add_e184c/2
  Subtract_36910/1 -> Product_6de9c/1
  Subtract_d1c76/1 -> Product_6de9c/2
  Product_11e1d/1 -> Add_e184c/1
  Product_6de9c/1 -> Divide_59545/1
  Constant_x_ddd_549c7/1 -> Divide_59545/2
  Add_e184c/1 -> Add_ac568/1
  Divide_59545/1 -> Add_ac568/2
  Add_ac568/1 -> Divide_0fc3d/1
  Constant_T_ddd_8ec66/1 -> Divide_0fc3d/2

== system case8/SG_D_3/d_psi_d_SG_D_3_block ==
  note: d_psi_d_SG_D_3 in case8
      | $2\,\pi \,f_{0}\,\left(v_{d,\mathrm{SG},D,3}\,\sin\left(\theta _{\mathrm{SG},D,3}\right)-v_{q,\mathrm{SG},D,3}\,\cos\left(\theta _{\mathrm{SG},D,3}\right)+\frac{R_{a}\,\left(\frac{\psi _{\mathrm{1d},\mathrm{SG},D,3}\,\left(x_{\mathrm{dd}}-x_{\mathrm{ddd}}\right)}{x_{\mathrm{dd}}-x_{l}}-\psi _{d,\mathrm{SG},D,3}+\frac{\psi _{\mathrm{fd},\mathrm{SG},D,3}\,\left(x_{\mathrm{ddd}}-x_{l}\right)}{x_{\mathrm{dd}}-x_{l}}\right)}{x_{\mathrm{ddd}}}+\frac{\psi _{q,\mathrm{SG},D,3}\,w_{\mathrm{SG},D,3}}{2\,f_{0}\,\pi }\right)$
      | Automatically generated on 2025-10-31 19:30:05 .
  State_psi_1d_SG_D_3_4ea1a : Inport
  State_psi_d_SG_D_3_63877 : Inport  Port=2
  State_psi_fd_SG_D_3_636d2 : Inport  Port=3
  Input_v_d_SG_D_3_0c684 : Inport  Port=4
  State_theta_SG_D_3_df685 : Inport  Port=5
  Input_v_q_SG_D_3_4be76 : Inport  Port=6
  State_theta_SG_D_3_0fee2 : Inport  Port=7
  State_psi_q_SG_D_3_c42a8 : Inport  Port=8
  State_w_SG_D_3_47940 : Inport  Port=9
  Add_92f12 : Sum
  Add_bd4ed : Sum
  Constant_-1_6d08d : Constant  Value=-1
  Constant_-2.0_8ac37 : Constant  Value=-2.0
  Constant_2.0_0fdc8 : Constant  Value=2.0
  Constant_R_a_5df35 : Constant  Value=R_a
  Constant_f0_0cbd7 : Constant  Value=f0
  Constant_f0_89302 : Constant  Value=f0
  Constant_pi_86fcd : Constant  Value=pi
  Constant_pi_bd109 : Constant  Value=pi
  Constant_x_dd_48013 : Constant  Value=x_dd
  Constant_x_dd_58d8a : Constant  Value=x_dd
  Constant_x_dd_bec6a : Constant  Value=x_dd
  Constant_x_ddd_7bb41 : Constant  Value=x_ddd
  Constant_x_ddd_b7800 : Constant  Value=x_ddd
  Constant_x_ddd_fdfcf : Constant  Value=x_ddd
  Constant_x_l_0f466 : Constant  Value=x_l
  Constant_x_l_3cf4b : Constant  Value=x_l
  Constant_x_l_fd86e : Constant  Value=x_l
  Divide_177c8 : Product  Inputs=*/
  Divide_2eedf : Product  Inputs=*/
  Divide_cf3a4 : Product  Inputs=*/
  Divide_e65b8 : Product  Inputs=*/
  MathFunc_cos_d4012 : Trigonometry  Operator=cos
  MathFunc_sin_8aebc : Trigonometry
  Product_10908 : Product
  Product_273be : Product
  Product_7b2ea : Product
  Product_80c4f : Product
  Product_99446 : Product
  Product_ad44f : Product
  Product_b39e8 : Product
  Product_d69ba : Product
  Product_e2610 : Product
  Product_e475d : Product
  Product_eaef2 : Product
  Product_f0187 : Product
  Subtract_406d3 : Sum  Inputs=+-
  Subtract_4ea41 : Sum  Inputs=+-
  Subtract_50f9b : Sum  Inputs=+-
  Subtract_9b616 : Sum  Inputs=+-
  Subtract_aef53 : Sum  Inputs=+-
  Subtract_e70a5 : Sum  Inputs=+-
  Subtract_fb5d1 : Sum  Inputs=+-
  Blockout_d_psi_d_SG_D_3_3f46c : Outport
  wires:
  Constant_-1_6d08d/1 -> Product_99446/1
  Constant_2.0_0fdc8/1 -> Product_80c4f/1
  Constant_x_dd_bec6a/1 -> Subtract_50f9b/1
  State_psi_1d_SG_D_3_4ea1a/1 -> Product_99446/2
  Constant_x_dd_48013/1 -> Subtract_4ea41/1
  Constant_pi_86fcd/1 -> Product_80c4f/2
  Constant_x_ddd_fdfcf/1 -> Subtract_50f9b/2
  Product_99446/1 -> Product_e2610/1
  Product_80c4f/1 -> Product_eaef2/1
  Subtract_50f9b/1 -> Product_e2610/2
  Constant_-2.0_8ac37/1 -> Product_b39e8/1
  Constant_x_l_0f466/1 -> Subtract_4ea41/2
  Constant_x_ddd_7bb41/1 -> Subtract_fb5d1/1
  Constant_pi_bd109/1 -> Product_b39e8/2
  Constant_x_l_fd86e/1 -> Subtract_fb5d1/2
  Product_f0187/1 -> Divide_cf3a4/1
  Product_e2610/1 -> Divide_177c8/1
  Subtract_4ea41/1 -> Divide_177c8/2
  State_psi_fd_SG_D_3_636d2/1 -> Product_10908/1
  Subtract_fb5d1/1 -> Product_10908/2
  Constant_x_dd_58d8a/1 -> Subtract_e70a5/1
  Constant_x_l_3cf4b/1 -> Subtract_e70a5/2
  Divide_cf3a4/1 -> Subtract_9b616/2
  Divide_177c8/1 -> Add_92f12/1
  Subtract_aef53/1 -> Product_7b2ea/2
  State_psi_d_SG_D_3_63877/1 -> Add_92f12/2
  Product_10908/1 -> Divide_2eedf/1
  Subtract_e70a5/1 -> Divide_2eedf/2
  Add_92f12/1 -> Subtract_aef53/1
  Divide_2eedf/1 -> Subtract_aef53/2
  Product_ad44f/1 -> Add_bd4ed/2
  Constant_R_a_5df35/1 -> Product_7b2ea/1
  Product_d69ba/1 -> Product_273be/1
  State_theta_SG_D_3_df685/1 -> MathFunc_sin_8aebc/1
  Product_7b2ea/1 -> Divide_e65b8/1
  Constant_x_ddd_b7800/1 -> Divide_e65b8/2
  Input_v_d_SG_D_3_0c684/1 -> Product_e475d/1
  State_w_SG_D_3_47940/1 -> Product_f0187/2
  MathFunc_sin_8aebc/1 -> Product_e475d/2
  State_theta_SG_D_3_0fee2/1 -> MathFunc_cos_d4012/1
  MathFunc_cos_d4012/1 -> Product_ad44f/2
  Divide_e65b8/1 -> Subtract_406d3/1
  Product_e475d/1 -> Subtract_406d3/2
  Input_v_q_SG_D_3_4be76/1 -> Product_ad44f/1
  State_psi_q_SG_D_3_c42a8/1 -> Product_f0187/1
  Constant_f0_0cbd7/1 -> Product_eaef2/2
  Subtract_406d3/1 -> Add_bd4ed/1
  Product_eaef2/1 -> Divide_cf3a4/2
  Product_b39e8/1 -> Product_d69ba/1
  Constant_f0_89302/1 -> Product_d69ba/2
  Add_bd4ed/1 -> Subtract_9b616/1
  Subtract_9b616/1 -> Product_273be/2
  Product_273be/1 -> Blockout_d_psi_d_SG_D_3_3f46c/1

== system case8/SG_D_3/d_psi_fd_SG_D_3_block ==
  note: d_psi_fd_SG_D_3 in case8
      | $-\frac{\psi _{\mathrm{fd},\mathrm{SG},D,3}-E_{\mathrm{fd},\mathrm{SG},D,3}+\left(x_{d}-x_{\mathrm{dd}}\right)\,\left(\frac{\frac{\psi _{\mathrm{1d},\mathrm{SG},D,3}\,\left(x_{\mathrm{dd}}-x_{\mathrm{ddd}}\right)}{x_{\mathrm{dd}}-x_{l}}-\psi _{d,\mathrm{SG},D,3}+\frac{\psi _{\mathrm{fd},\mathrm{SG},D,3}\,\left(x_{\mathrm{ddd}}-x_{l}\right)}{x_{\mathrm{dd}}-x_{l}}}{x_{\mathrm{ddd}}}-\frac{\left(x_{\mathrm{dd}}-x_{\mathrm{ddd}}\right)\,\left(\psi _{\mathrm{1d},\mathrm{SG},D,3}-\psi _{\mathrm{fd},\mathrm{SG},D,3}+\frac{\left(x_{\mathrm{dd}}-x_{l}\right)\,\left(\frac{\psi _{\mathrm{1d},\mathrm{SG},D,3}\,\left(x_{\mathrm{dd}}-x_{\mathrm{ddd}}\right)}{x_{\mathrm{dd}}-x_{l}}-\psi _{d,\mathrm{SG},D,3}+\frac{\psi _{\mathrm{fd},\mathrm{SG},D,3}\,\left(x_{\mathrm{ddd}}-x_{l}\right)}{x_{\mathrm{dd}}-x_{l}}\right)}{x_{\mathrm{ddd}}}\right)}{{\left(x_{\mathrm{dd}}-x_{l}\right)}^2}\right)}{T_{\mathrm{dd}}}$
      | Automatically generated on 2025-10-31 19:30:08 .
  State_E_fd_SG_D_3_14ff0 : Inport
  State_psi_fd_SG_D_3_191f5 : Inport  Port=2
  State_psi_1d_SG_D_3_ed615 : Inport  Port=3
  State_psi_fd_SG_D_3_b9793 : Inport  Port=4
  State_psi_1d_SG_D_3_498fb : Inport  Port=5
  State_psi_d_SG_D_3_275f4 : Inport  Port=6
  State_psi_fd_SG_D_3_7365a : Inport  Port=7
  State_psi_1d_SG_D_3_b1cc2 : Inport  Port=8
  State_psi_d_SG_D_3_8cb70 : Inport  Port=9
  State_psi_fd_SG_D_3_47206 : Inport  Port=10
  Add_03380 : Sum
  Add_e91d6 : Sum
  Constant_-1_2bbfc : Constant  Value=-1
  Constant_-1_bc540 : Constant  Value=-1
  Constant_-1_dc14b : Constant  Value=-1
  Constant_2.0_ad7e8 : Constant  Value=2.0
  Constant_T_dd_9c4d7 : Constant  Value=T_dd
  Constant_x_d_2e69f : Constant  Value=x_d
  Constant_x_dd_25bf1 : Constant  Value=x_dd
  Constant_x_dd_579b5 : Constant  Value=x_dd
  Constant_x_dd_64b76 : Constant  Value=x_dd
  Constant_x_dd_83074 : Constant  Value=x_dd
  Constant_x_dd_b129e : Constant  Value=x_dd
  Constant_x_dd_cd2f2 : Constant  Value=x_dd
  Constant_x_dd_def97 : Constant  Value=x_dd
  Constant_x_dd_ed2f5 : Constant  Value=x_dd
  Constant_x_dd_ed4f9 : Constant  Value=x_dd
  Constant_x_dd_f7ad5 : Constant  Value=x_dd
  Constant_x_ddd_48dab : Constant  Value=x_ddd
  Constant_x_ddd_79b82 : Constant  Value=x_ddd
  Constant_x_ddd_82bc3 : Constant  Value=x_ddd
  Constant_x_ddd_8f481 : Constant  Value=x_ddd
  Constant_x_ddd_aaf03 : Constant  Value=x_ddd
  Constant_x_ddd_c9660 : Constant  Value=x_ddd
  Constant_x_ddd_f25a2 : Constant  Value=x_ddd
  Constant_x_l_12b34 : Constant  Value=x_l
  Constant_x_l_16263 : Constant  Value=x_l
  Constant_x_l_3c9ab : Constant  Value=x_l
  Constant_x_l_63e6a : Constant  Value=x_l
  Constant_x_l_b5cb1 : Constant  Value=x_l
  Constant_x_l_b8257 : Constant  Value=x_l
  Constant_x_l_e2690 : Constant  Value=x_l
  Constant_x_l_fa24a : Constant  Value=x_l
  Divide_01045 : Product  Inputs=*/
  Divide_22899 : Product  Inputs=*/
  Divide_2d66b : Product  Inputs=*/
  Divide_85e2e : Product  Inputs=*/
  Divide_860bd : Product  Inputs=*/
  Divide_c8e74 : Product  Inputs=*/
  Divide_cb57c : Product  Inputs=*/
  Divide_f9be5 : Product  Inputs=*/
  Power_f7f57 : Math  Operator=pow
  Product_04c7d : Product
  Product_23130 : Product
  Product_34239 : Product
  Product_45993 : Product
  Product_4890b : Product
  Product_4c6f7 : Product
  Product_52bd2 : Product
  Product_b3329 : Product
  Product_eddb2 : Product
  Product_f8e5c : Product
  Subtract_11f2e : Sum  Inputs=+-
  Subtract_1a41e : Sum  Inputs=+-
  Subtract_1d3c5 : Sum  Inputs=+-
  Subtract_243f5 : Sum  Inputs=+-
  Subtract_36f42 : Sum  Inputs=+-
  Subtract_39669 : Sum  Inputs=+-
  Subtract_47fc9 : Sum  Inputs=+-
  Subtract_52348 : Sum  Inputs=+-
  Subtract_56b0d : Sum  Inputs=+-
  Subtract_5e0af : Sum  Inputs=+-
  Subtract_829f1 : Sum  Inputs=+-
  Subtract_a1ac9 : Sum  Inputs=+-
  Subtract_bd3ed : Sum  Inputs=+-
  Subtract_c12ed : Sum  Inputs=+-
  Subtract_c78e7 : Sum  Inputs=+-
  Subtract_d05a4 : Sum  Inputs=+-
  Subtract_d0dc1 : Sum  Inputs=+-
  Subtract_e8b12 : Sum  Inputs=+-
  Subtract_eed67 : Sum  Inputs=+-
  Blockout_d_psi_fd_SG_D_3_efa73 : Outport
  wires:
  Product_eddb2/1 -> Divide_f9be5/1
  Constant_-1_2bbfc/1 -> Product_23130/1
  Subtract_11f2e/1 -> Product_4890b/2
  State_psi_1d_SG_D_3_498fb/1 -> Product_23130/2
  Constant_x_l_63e6a/1 -> Subtract_e8b12/2
  Constant_x_dd_cd2f2/1 -> Subtract_11f2e/1
  Constant_x_ddd_c9660/1 -> Subtract_11f2e/2
  Product_23130/1 -> Product_4890b/1
  Constant_x_dd_25bf1/1 -> Subtract_d0dc1/1
  Constant_x_l_fa24a/1 -> Subtract_d0dc1/2
  Constant_x_ddd_79b82/1 -> Subtract_eed67/2
  Constant_x_ddd_f25a2/1 -> Subtract_d05a4/1
  Constant_x_l_3c9ab/1 -> Subtract_d05a4/2
  Product_34239/1 -> Product_4c6f7/1
  Product_4890b/1 -> Divide_cb57c/1
  Subtract_d0dc1/1 -> Divide_cb57c/2
  State_psi_fd_SG_D_3_7365a/1 -> Product_45993/1
  Constant_x_ddd_aaf03/1 -> Subtract_e8b12/1
  Subtract_d05a4/1 -> Product_45993/2
  Constant_x_dd_ed2f5/1 -> Subtract_829f1/1
  Constant_-1_bc540/1 -> Product_34239/1
  Constant_x_l_e2690/1 -> Subtract_829f1/2
  Product_4c6f7/1 -> Divide_01045/1
  Divide_cb57c/1 -> Add_03380/1
  Product_f8e5c/1 -> Divide_22899/1
  State_psi_d_SG_D_3_275f4/1 -> Add_03380/2
  State_psi_fd_SG_D_3_47206/1 -> Product_f8e5c/1
  Product_45993/1 -> Divide_860bd/1
  Constant_x_dd_64b76/1 -> Subtract_47fc9/1
  Subtract_829f1/1 -> Divide_860bd/2
  Constant_x_l_12b34/1 -> Subtract_56b0d/2
  Constant_x_dd_b129e/1 -> Subtract_c78e7/1
  Subtract_bd3ed/1 -> Product_b3329/2
  Constant_x_l_b8257/1 -> Subtract_c78e7/2
  Divide_01045/1 -> Add_e91d6/1
  Constant_x_ddd_48dab/1 -> Divide_f9be5/2
  Add_03380/1 -> Subtract_5e0af/1
  Divide_860bd/1 -> Subtract_5e0af/2
  State_psi_1d_SG_D_3_b1cc2/1 -> Product_34239/2
  Constant_x_l_b5cb1/1 -> Subtract_47fc9/2
  Constant_x_dd_579b5/1 -> Subtract_eed67/1
  Subtract_c78e7/1 -> Product_eddb2/1
  Add_e91d6/1 -> Subtract_36f42/1
  Subtract_5e0af/1 -> Product_eddb2/2
  Subtract_eed67/1 -> Product_4c6f7/2
  Constant_x_dd_ed4f9/1 -> Subtract_1a41e/1
  Constant_x_l_16263/1 -> Subtract_1a41e/2
  Subtract_e8b12/1 -> Product_f8e5c/2
  Constant_x_dd_def97/1 -> Subtract_bd3ed/1
  Constant_x_ddd_82bc3/1 -> Subtract_bd3ed/2
  Product_b3329/1 -> Product_52bd2/1
  State_psi_1d_SG_D_3_ed615/1 -> Subtract_c12ed/1
  Subtract_1a41e/1 -> Divide_01045/2
  State_psi_fd_SG_D_3_b9793/1 -> Subtract_c12ed/2
  Constant_-1_dc14b/1 -> Product_b3329/1
  Subtract_c12ed/1 -> Subtract_52348/1
  Divide_f9be5/1 -> Subtract_52348/2
  Constant_x_dd_f7ad5/1 -> Subtract_56b0d/1
  Divide_22899/1 -> Subtract_36f42/2
  State_psi_d_SG_D_3_8cb70/1 -> Add_e91d6/2
  Subtract_47fc9/1 -> Divide_22899/2
  Subtract_52348/1 -> Product_52bd2/2
  Subtract_56b0d/1 -> Power_f7f57/1
  Constant_2.0_ad7e8/1 -> Power_f7f57/2
  Product_52bd2/1 -> Divide_c8e74/1
  Subtract_a1ac9/1 -> Product_04c7d/2
  Power_f7f57/1 -> Divide_c8e74/2
  Subtract_36f42/1 -> Divide_2d66b/1
  Constant_x_ddd_8f481/1 -> Divide_2d66b/2
  Constant_x_d_2e69f/1 -> Subtract_39669/1
  Constant_x_dd_83074/1 -> Subtract_39669/2
  Divide_c8e74/1 -> Subtract_a1ac9/1
  Divide_2d66b/1 -> Subtract_a1ac9/2
  State_E_fd_SG_D_3_14ff0/1 -> Subtract_1d3c5/1
  State_psi_fd_SG_D_3_191f5/1 -> Subtract_1d3c5/2
  Subtract_39669/1 -> Product_04c7d/1
  Subtract_1d3c5/1 -> Subtract_243f5/1
  Product_04c7d/1 -> Subtract_243f5/2
  Subtract_243f5/1 -> Divide_85e2e/1
  Constant_T_dd_9c4d7/1 -> Divide_85e2e/2
  Divide_85e2e/1 -> Blockout_d_psi_fd_SG_D_3_efa73/1
